simulink model "converter_uniqueness"  (R2015b)
settings: Solver=VariableStepAuto  StartTime=0.0  StopTime=100*T_mach  RelTol=1e-3
values from neighbouring files (symbols this model uses):
  c2_val = (1-V_ref/Vd_val)/(8*v2_ripple*l2_val*f_sw^2)    (= 0.0001)    [PowerSupplyScript.m]    (also in master_conv.m; master_conv2.m; matlab.mat = 1e-05; normal_buck_comparison.m = 1e-05)
  f_sw = 50e3    (= 50000)    [PowerSupplyScript.m]    (also in master_conv.m; master_conv2.m; matlab.mat)
  l1_val = Vo1*(Vd_val-Vo1)/(delta_i1*f_sw*Vd_val)    (= 0.00181818181818)    [PowerSupplyScript.m]    (also in master_conv.m = 0.000181818181818; master_conv2.m; matlab.mat; poles_locus.m = l1_val_bak)
  r_val = 1    [PowerSupplyScript.m]    (also in master_conv.m; master_conv2.m; matlab.mat)
  rc2_val = 0.0001    [PowerSupplyScript.m]    (also in master_conv.m; master_conv2.m; matlab.mat)
  rl1_val = 0.0002    [PowerSupplyScript.m]    (also in master_conv.m; master_conv2.m; matlab.mat)
  Vd_val = 110    [PowerSupplyScript.m]    (also in master_conv.m; master_conv2.m; matlab.mat)
libraries: powerlib x29
settings Model: Creator=akshay  LastModifiedBy=akshay

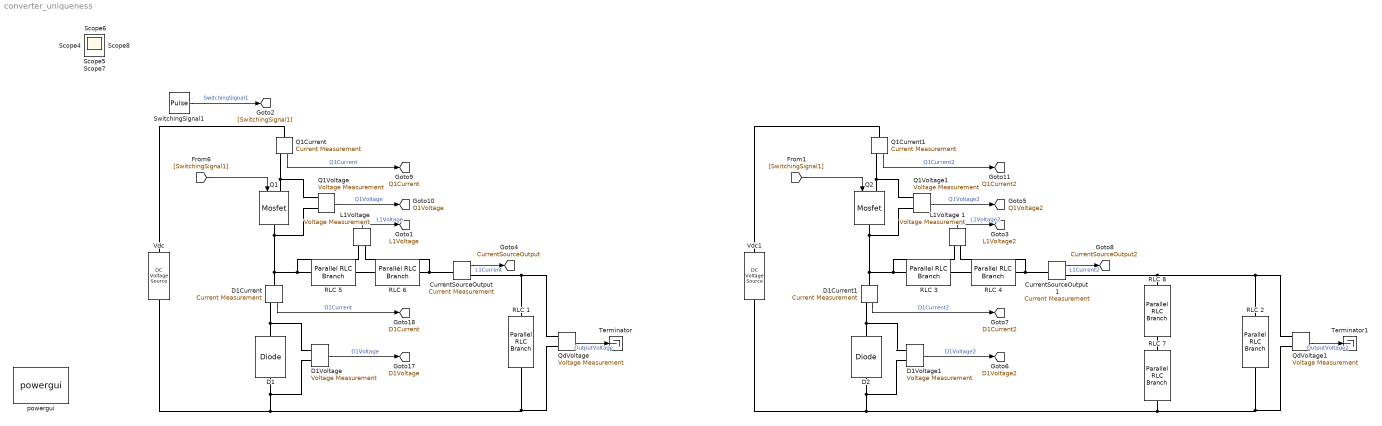
== system converter_uniqueness ==
  " RLC 1" : powerlib/Elements/Parallel RLC Branch  LConnTagsString=a  RConnTagsString=__new0  BranchType=R  Resistance=r_val  Inductance=1e-3  SetiL0=off  InitialCurrent=0  Capacitance=0.1e-6  Setx0=off  InitialVoltage=0  Measurements=None
  " RLC 2" : powerlib/Elements/Parallel RLC Branch  LConnTagsString=a  RConnTagsString=__new0  BranchType=R  Resistance=r_val  Inductance=1e-3  SetiL0=off  InitialCurrent=0  Capacitance=0.1e-6  Setx0=off  InitialVoltage=0  Measurements=None
  " RLC 3" : powerlib/Elements/Parallel RLC Branch  LConnTagsString=a  RConnTagsString=__new0  BranchType=R  Resistance=rl1_val  Inductance=5e-6  SetiL0=off  InitialCurrent=0  Capacitance=0.3e-6  Setx0=off  InitialVoltage=0  Measurements=None
  " RLC 4" : powerlib/Elements/Parallel RLC Branch  LConnTagsString=a  RConnTagsString=__new0  BranchType=L  Resistance=50  Inductance=l1_val  SetiL0=off  InitialCurrent=100  Capacitance=0.3e-6  Setx0=off  InitialVoltage=0  Measurements=None
  " RLC 5" : powerlib/Elements/Parallel RLC Branch  LConnTagsString=a  RConnTagsString=__new0  BranchType=R  Resistance=rl1_val  Inductance=5e-6  SetiL0=off  InitialCurrent=0  Capacitance=0.3e-6  Setx0=off  InitialVoltage=0  Measurements=None
  " RLC 6" : powerlib/Elements/Parallel RLC Branch  LConnTagsString=a  RConnTagsString=__new0  BranchType=L  Resistance=50  Inductance=l1_val  SetiL0=off  InitialCurrent=100  Capacitance=0.3e-6  Setx0=off  InitialVoltage=0  Measurements=None
  " RLC 7" : powerlib/Elements/Parallel RLC Branch  LConnTagsString=a  RConnTagsString=__new0  BranchType=C  Resistance=1  Inductance=1e-3  SetiL0=off  InitialCurrent=0  Capacitance=c2_val  Setx0=off  InitialVoltage=50  Measurements=None
  " RLC 8" : powerlib/Elements/Parallel RLC Branch  LConnTagsString=a  RConnTagsString=__new0  BranchType=R  Resistance=rc2_val  Inductance=1e-3  SetiL0=off  InitialCurrent=0  Capacitance=0.1e-6  Setx0=off  InitialVoltage=0  Measurements=None
  CurrentSourceOutput : powerlib/Measurements/Current Measurement  PhasorSimulation=off  OutputType=Complex  PSBequivalent=0
  CurrentSourceOutput1 : powerlib/Measurements/Current Measurement  PhasorSimulation=off  OutputType=Complex  PSBequivalent=0
  D1 : powerlib/Power Electronics/Diode  Ron=0.001  Lon=0  Vf=0.8  IC=0  UseSnubber=off  Rs=1e5  Cs=250e-9  Measurements=off
  D1Current : powerlib/Measurements/Current Measurement  PhasorSimulation=off  OutputType=Complex  PSBequivalent=0
  D1Current1 : powerlib/Measurements/Current Measurement  PhasorSimulation=off  OutputType=Complex  PSBequivalent=0
  D1Voltage : powerlib/Measurements/Voltage Measurement  PhasorSimulation=off  OutputType=Complex  PSBequivalent=0
  D1Voltage1 : powerlib/Measurements/Voltage Measurement  PhasorSimulation=off  OutputType=Complex  PSBequivalent=0
  D2 : powerlib/Power Electronics/Diode  Ron=0.001  Lon=0  Vf=0.8  IC=0  UseSnubber=off  Rs=1e5  Cs=250e-9  Measurements=off
  "L1Voltage " : powerlib/Measurements/Voltage Measurement  PhasorSimulation=off  OutputType=Complex  PSBequivalent=0
  L1Voltage 1 : powerlib/Measurements/Voltage Measurement  PhasorSimulation=off  OutputType=Complex  PSBequivalent=0
  Q1 : powerlib/Power Electronics/Mosfet  Ron=0.1  Lon=0  Rd=0.01  Vfd=0  IC=0  Rs=1e5  Cs=inf  Measurements=off
  Q1Current : powerlib/Measurements/Current Measurement  PhasorSimulation=off  OutputType=Complex  PSBequivalent=0
  Q1Current1 : powerlib/Measurements/Current Measurement  PhasorSimulation=off  OutputType=Complex  PSBequivalent=0
  Q1Voltage : powerlib/Measurements/Voltage Measurement  PhasorSimulation=off  OutputType=Complex  PSBequivalent=0
  Q1Voltage1 : powerlib/Measurements/Voltage Measurement  PhasorSimulation=off  OutputType=Complex  PSBequivalent=0
  Q2 : powerlib/Power Electronics/Mosfet  Ron=0.1  Lon=0  Rd=0.01  Vfd=0  IC=0  Rs=1e5  Cs=inf  Measurements=off
  QdVoltage : powerlib/Measurements/Voltage Measurement  PhasorSimulation=off  OutputType=Complex  PSBequivalent=0
  QdVoltage1 : powerlib/Measurements/Voltage Measurement  PhasorSimulation=off  OutputType=Complex  PSBequivalent=0
  SwitchingSignal1 : DiscretePulseGenerator  PulseType=Time based  Period=1/f_sw  PulseWidth=20
  Terminator : Terminator
  Terminator1 : Terminator
  Vdc : powerlib/Electrical Sources/DC Voltage Source  Amplitude=Vd_val  Measurements=Voltage
  Vdc1 : powerlib/Electrical Sources/DC Voltage Source  Amplitude=Vd_val  Measurements=Voltage
  powergui : powerlib/powergui  Priority=1  SimulationMode=Discrete  SolverType=Backward Euler  SampleTime=0.01/f_sw  frequency=60  SPID=on  DisableSnubberDevices=off  DisableRonSwitches=off  DisableVfSwitches=off  SwTol=0  DisplayEquations=off  Interpol=off  ExternalGateDelay=off  methode=off  Ts=0  FunctionMessages=off  echomessages=off  HookPort=off  EnableUseOfTLC=off  x0status=zero  frequencyindice=0  Pbase=100e6  ErrMax=1e-4  Iterations=50  UnitsV=kV  UnitsW=MW  buscounter=0  RestoreLinks=warning  ResistiveCurrentMeasurement=off  Frange=[0:2:500]  Ylog=off  Xlog=on  ShowGrid=off  save=off  variable=ZData  structure=ScopeData  ZoomFFT=off  StartTime=0.0  cycles=5  DisplayStyle=2  fundamental=50  FreqAxis=off  MaxFrequency=50000  frequencyindicesteady=1  RmsSteady=1  display=off
  Scope{,1..8} (9 alike) : Scope
  tag scope: CurrentSourceOutput2=global, CurrentSourceOutput=global, D1Current2=global, D1Current=global, D1Voltage2=global, D1Voltage=global, L1Voltage2=global, L1Voltage=global, Q1Current2=global, Q1Current=global, Q1Voltage2=global, Q1Voltage=global
  wires:
  CurrentSourceOutput/1 -> [CurrentSourceOutput]  "L1Current"
  [SwitchingSignal1] -> Q1/1
  Q1Current/1 -> [Q1Current]  "Q1Current"
  Q1Voltage/1 -> [Q1Voltage]  "Q1Voltage"
  D1Current/1 -> [D1Current]  "D1Current"
  D1Voltage/1 -> [D1Voltage]  "D1Voltage"
  "L1Voltage "/1 -> [L1Voltage]  "L1Voltage"
  SwitchingSignal1/1 -> [SwitchingSignal1]  "SwitchingSignal1"
  QdVoltage/1 -> Terminator/1  "OutputVoltage"
  CurrentSourceOutput1/1 -> [CurrentSourceOutput2]  "L1Current2"
  [SwitchingSignal1] -> Q2/1
  Q1Current1/1 -> [Q1Current2]  "Q1Current2"
  Q1Voltage1/1 -> [Q1Voltage2]  "Q1Voltage2"
  D1Current1/1 -> [D1Current2]  "D1Current2"
  D1Voltage1/1 -> [D1Voltage2]  "D1Voltage2"
  L1Voltage 1/1 -> [L1Voltage2]  "L1Voltage2"
  QdVoltage1/1 -> Terminator1/1  "OutputVoltage2"
  connections:
  Q1/RConn1 -- D1Current/LConn1 -- "L1Voltage "/LConn1 -- " RLC 5"/LConn1 -- Q1Voltage/LConn2
  " RLC 6"/RConn1 -- CurrentSourceOutput/LConn1 -- "L1Voltage "/LConn2
  Q1/LConn1 -- Q1Current/RConn1 -- Q1Voltage/LConn1
  D1Voltage/LConn1 -- D1Current/RConn1 -- D1/RConn1
  D1/LConn1 -- D1Voltage/LConn2 -- Vdc/LConn1 -- QdVoltage/LConn2 -- " RLC 1"/RConn1
  Vdc/RConn1 -- Q1Current/LConn1
  " RLC 5"/RConn1 -- " RLC 6"/LConn1
  CurrentSourceOutput/RConn1 -- " RLC 1"/LConn1 -- QdVoltage/LConn1
  Q2/RConn1 -- Q1Voltage1/LConn2 -- D1Current1/LConn1 -- L1Voltage 1/LConn1 -- " RLC 3"/LConn1
  " RLC 4"/RConn1 -- CurrentSourceOutput1/LConn1 -- L1Voltage 1/LConn2
  Q2/LConn1 -- Q1Current1/RConn1 -- Q1Voltage1/LConn1
  D1Voltage1/LConn1 -- D1Current1/RConn1 -- D2/RConn1
  D2/LConn1 -- D1Voltage1/LConn2 -- Vdc1/LConn1 -- " RLC 7"/RConn1 -- QdVoltage1/LConn2 -- " RLC 2"/RConn1
  QdVoltage1/LConn1 -- " RLC 8"/LConn1 -- CurrentSourceOutput1/RConn1 -- " RLC 2"/LConn1
  " RLC 3"/RConn1 -- " RLC 4"/LConn1
  Vdc1/RConn1 -- Q1Current1/LConn1
  " RLC 7"/LConn1 -- " RLC 8"/RConn1
